simulink model "IEEE13_ltc"  (Simulink 8.5)
settings: Solver=ode5  SolverMode=SingleTasking  StartTime=0.0  StopTime=86400  FixedStep=Ts  RelTol=1e-3
PostLoadFcn:
  | Ts=3;
InitFcn:
  | Ts=3;
libraries: simulink x5, rtlab x1, rtlab_phasor x1
settings Model: Creator=GunaBharati  LastModifiedBy=Jaimie.Swartz
settings DataIOCC: SignalLoggingSaveFormat=Dataset  SaveOutput=off  SaveTime=off
settings OptimizationCC: BlockReduction=off  OptimizeBlockIOStorage=off  BufferReuse=off  GlobalBufferReuse=off  ExpressionFolding=off  ExpressionDepthLimit=128  LocalBlockOutputs=off
settings DebuggingCC: UnderspecifiedInitializationDetection=Simplified  MergeDetectMultiDrivingBlocksExec=error  FcnCallInpInsideContextMsg=EnableAllAsError  StateNameClashWarn=none
settings GRTTargetCC: CombineOutputUpdateFcns=on  GRTInterface=off
settings ConfigurationSet: Description=SimMechanics 2G

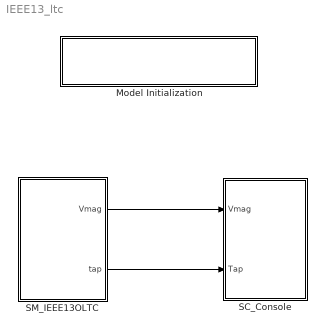
== system IEEE13_ltc ==
  Model Initialization : Subsystem  AncestorBlock=artemis/Tools /Misc/Model Initialization  mask(Model Functions){InitFcnX=Ts=3;, prel=off, posl=on, inif=on, strf=off}
      mask prompts: InitFcnX "Initialisation"; prel "Preload Function"; posl "PostLoad Function"; inif "InitFcn"; strf "StartFcn"
      mask init:
      | currentBlock = gcb;
      | root = bdroot(currentBlock);
      | 
      | if ~strcmp(get_param(root,'BlockDiagramType'),'library')
      |     if prel==1
      |         set_param(root, 'PreLoadFcn', InitFcnX);
      |     else
      |         set_param(root, 'PreLoadFcn', '');
      |     end
      |     if inif==1
      |         set_param(root, 'InitFcn', InitFcnX);
      |     else
      |         set_param(root, 'InitFcn', '');
      |     end
      |     if strf==1
      |         set_param(root, 'StartFcn', InitFcnX);
      |     else
      |         set_param(root, 'StartFcn', '');
      |     end
      |     if posl==1
      |         set_param(root, 'PostLoadFcn', InitFcnX);
      |     else
      |         set_param(root, 'PostLoadFcn', '');
      |     end
      | end
      | 
      | pos = get_param(currentBlock, 'Position');
      | width = pos(3) - pos(1); height = pos(4) - pos(2);
      | txt = [ upper(root) '\n' '- InitFcn. . . . . '  get_param(root, 'InitFcn') ];
      settings: CopyFcn=set_param(gcb,'LinkStatus','inactive')
      mask Display: text(5, height*0.5, txt, 'horizontalAlignment', 'left', 'verticalAlignment', 'middle') ;
  SC_Console : Subsystem
  SM_IEEE13OLTC : Subsystem
  wires:
  SM_IEEE13OLTC/1(Vmag) -> SC_Console/1(Vmag)
  SM_IEEE13OLTC/2(tap) -> SC_Console/2(Tap)

== system IEEE13_ltc/Model Initialization ==

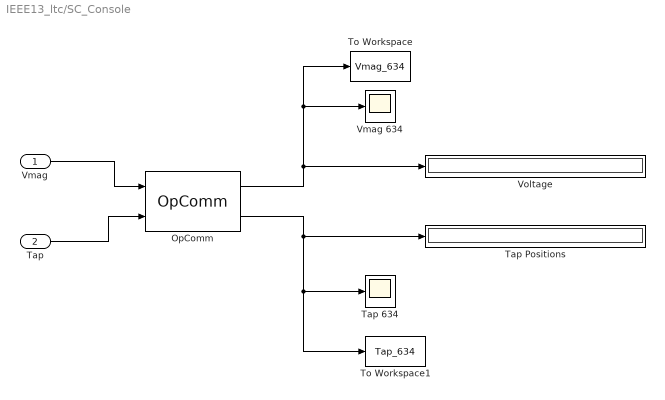
== system IEEE13_ltc/SC_Console ==
  Vmag : Inport
  Tap : Inport  Port=2
  OpComm : rtlab/OpComm  nbport=2  groupe_acq=1  subsys_rate=0  st=0  Synchronization=on  Interpolation=on  Threshold=1.0  Missed_Data=off  Sim_Time=off  Samples=off  dynSigOut=off  from_console=0  warning_done=off  writeOpCommFile=off  Offset=off
  Tap 634 : Scope
      settings: TimeRange=300  YMin=-1  YMax=1
  Tap Positions : Display
  To Workspace : ToWorkspace  VariableName=Vmag_634  SampleTime=-1
  To Workspace1 : ToWorkspace  VariableName=Tap_634  SampleTime=-1
  Vmag 634 : Scope
      settings: YMin=246.783  YMax=272.761
  Voltage : Display
  wires:
  Vmag/1 -> OpComm/1
  Tap/1 -> OpComm/2
  OpComm/1 -> Voltage/1, To Workspace/1, Vmag 634/1
  OpComm/2 -> Tap Positions/1, To Workspace1/1, Tap 634/1

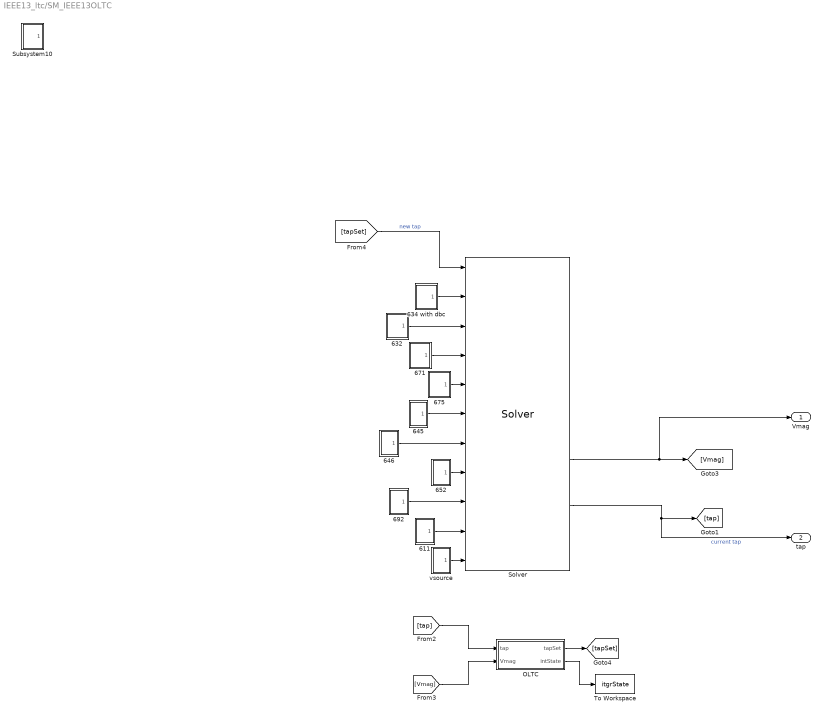
== system IEEE13_ltc/SM_IEEE13OLTC ==
  611 : Subsystem
  632 : Subsystem
  634 with dbc : Subsystem
  645 : Subsystem
  646 : Subsystem
  652 : Subsystem
  671 : Subsystem
  675 : Subsystem
  692 : Subsystem
  OLTC : Subsystem  mask{vRef=[260 260 260], intgConst=1200, deadBand=3.5/260, tapPos=[16 -16]}
      mask prompts: vRef "Reference Voltage: [a b c] voltage"; intgConst "Integrator Reset Value"; deadBand "Total Dead Band (pu)"; tapPos "[Max Min] Tap Positions"
      mask DialogControl DescTextVar Prompt: 3-Phase Voltage Regulator: Individual phase regulation enabled
  Solver : rtlab_phasor/Solver  epname=System  extension=Excel  xls='IEEE13_ltc_liz.xls'  raw='4992b.raw'  dyr='4992b.dyr'  cyme='typical.sxst'  powerfactory='network.dgs'  builtin=on  cyme_pf=''  cyme_unbalanced=on  lazy_netlist=off  capidir='CAPI'  fmudir=''  capiprefix=capicomp_  fmuprefix=fmucomp_  logging=off  sim_mode=Dynamic simulation only (without power-flow)  pf_max_it=100  pf_tol_v=0.00000001  pf_flat_start=off  pf_smart_start=off  pf_export=on  np=1  exporty=off  dt=Ts  optim_threads=on  perflog_on=off  script_activate_postinit=off  script_postinit_name=''
  Subsystem10 : Subsystem
  To Workspace : ToWorkspace  VariableName=itgrState  SampleTime=-1
  vsource : Subsystem
  Vmag : Outport
  tap : Outport  Port=2
  wires:
  Solver/5 -> Vmag/1, [Vmag]
  Solver/6 -> tap/1, [tap]  "current tap"
  OLTC/1(tapSet) -> [tapSet]
  [tapSet] -> Solver/1  "new tap"
  [Vmag] -> OLTC/2(Vmag)
  [tap] -> OLTC/1(tap)
  OLTC/2(intState) -> To Workspace/1
  632/1(Out1) -> Solver/3
  634 with dbc/1(Out1) -> Solver/2
  vsource/1(Out1) -> Solver/11
  611/1(Out1) -> Solver/10
  692/1(Out1) -> Solver/9
  652/1(Out1) -> Solver/8
  646/1(Out1) -> Solver/7
  645/1(Out1) -> Solver/6
  675/1(Out1) -> Solver/5
  671/1(Out1) -> Solver/4

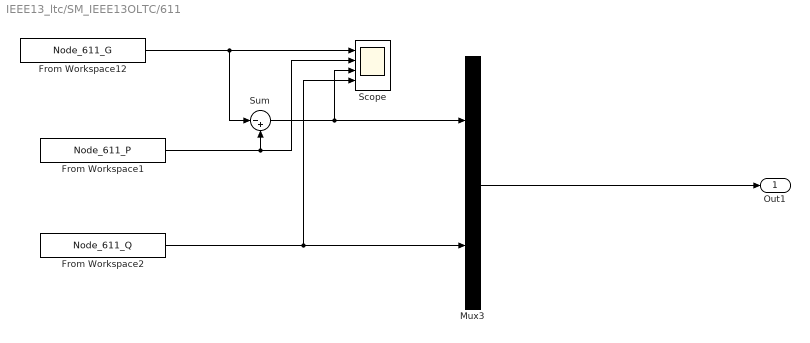
== system IEEE13_ltc/SM_IEEE13OLTC/611 ==
  From Workspace1 : FromWorkspace  VariableName=Node_611_P  SampleTime=Ts  OutputAfterFinalValue=Holding final value
  From Workspace12 : FromWorkspace  VariableName=Node_611_G  SampleTime=Ts  OutputAfterFinalValue=Holding final value
  From Workspace2 : FromWorkspace  VariableName=Node_611_Q  SampleTime=Ts  OutputAfterFinalValue=Holding final value
  Mux3 : Mux  Inputs=2
  Scope : Scope  NumInputPorts=4
      settings: YMin=229~-50~-5~-5  YMax=231~800~5~5  SampleInput=on  SampleTime=Ts
  Sum : Sum  Inputs=|-+
  Out1 : Outport
  wires:
  Mux3/1 -> Out1/1
  From Workspace2/1 -> Scope/4, Mux3/2
  From Workspace12/1 -> Sum/1, Scope/1
  Sum/1 -> Scope/3, Mux3/1
  From Workspace1/1 -> Sum/2, Scope/2

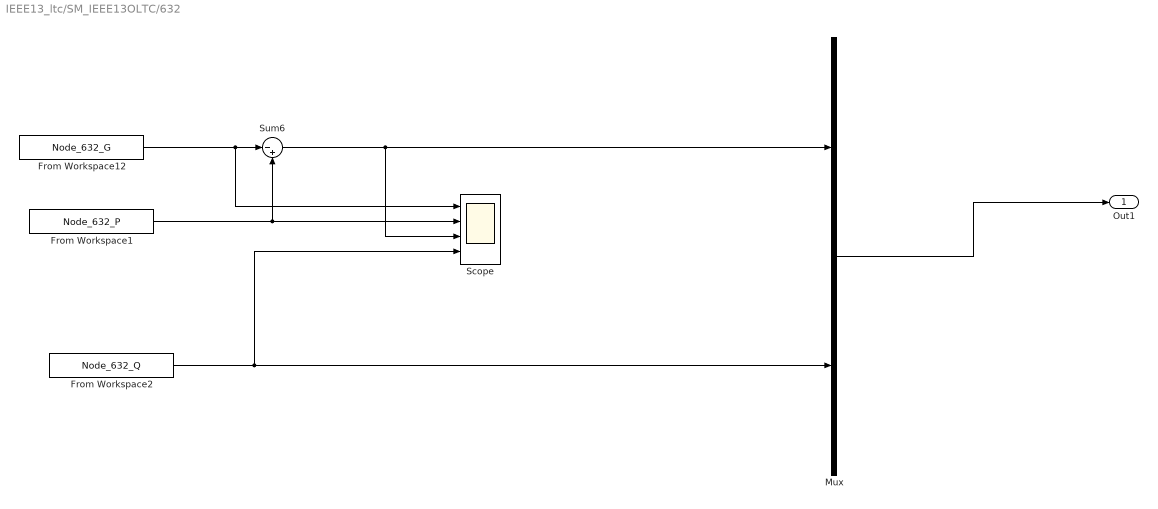
== system IEEE13_ltc/SM_IEEE13OLTC/632 ==
  From Workspace1 : FromWorkspace  VariableName=Node_632_P  SampleTime=Ts  OutputAfterFinalValue=Holding final value
  From Workspace12 : FromWorkspace  VariableName=Node_632_G  SampleTime=Ts  OutputAfterFinalValue=Holding final value
  From Workspace2 : FromWorkspace  VariableName=Node_632_Q  SampleTime=Ts  OutputAfterFinalValue=Holding final value
  Mux : Mux  Inputs=2
  Scope : Scope  NumInputPorts=4
      settings: YMin=229~-50~-5~-5  YMax=231~800~5~5  SaveName=ScopeData2  SampleInput=on  SampleTime=Ts
  Sum6 : Sum  Inputs=|-+
  Out1 : Outport
  wires:
  Mux/1 -> Out1/1
  From Workspace2/1 -> Mux/2, Scope/4
  From Workspace12/1 -> Scope/1, Sum6/1
  Sum6/1 -> Scope/3, Mux/1
  From Workspace1/1 -> Sum6/2, Scope/2

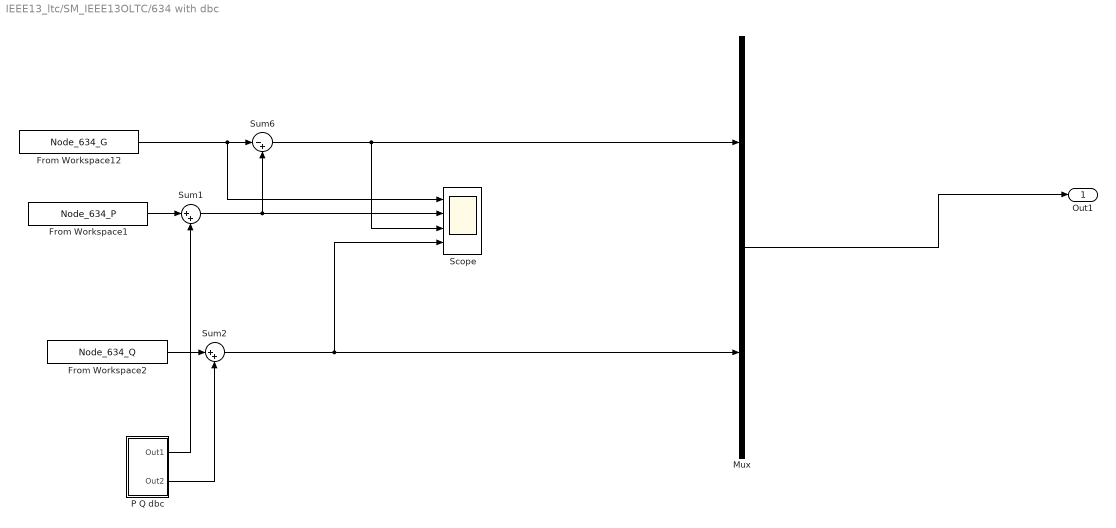
== system IEEE13_ltc/SM_IEEE13OLTC/634 with dbc ==
  From Workspace1 : FromWorkspace  VariableName=Node_634_P  SampleTime=Ts  OutputAfterFinalValue=Holding final value
  From Workspace12 : FromWorkspace  VariableName=Node_634_G  SampleTime=Ts  OutputAfterFinalValue=Holding final value
  From Workspace2 : FromWorkspace  VariableName=Node_634_Q  SampleTime=Ts  OutputAfterFinalValue=Holding final value
  Mux : Mux  Inputs=2
  P Q dbc : Subsystem
  Scope : Scope  NumInputPorts=4
      settings: YMin=229~-50~-5~-5  YMax=231~800~5~5  SaveName=ScopeData2  SampleInput=on  SampleTime=Ts
  Sum1 : Sum  Inputs=|++
  Sum2 : Sum  Inputs=|++
  Sum6 : Sum  Inputs=|-+
  Out1 : Outport
  wires:
  Mux/1 -> Out1/1
  From Workspace12/1 -> Scope/1, Sum6/1
  Sum6/1 -> Scope/3, Mux/1
  From Workspace1/1 -> Sum1/1
  Sum1/1 -> Sum6/2, Scope/2
  Sum2/1 -> Mux/2, Scope/4
  From Workspace2/1 -> Sum2/1
  P Q dbc/2(Out2) -> Sum2/2
  P Q dbc/1(Out1) -> Sum1/2

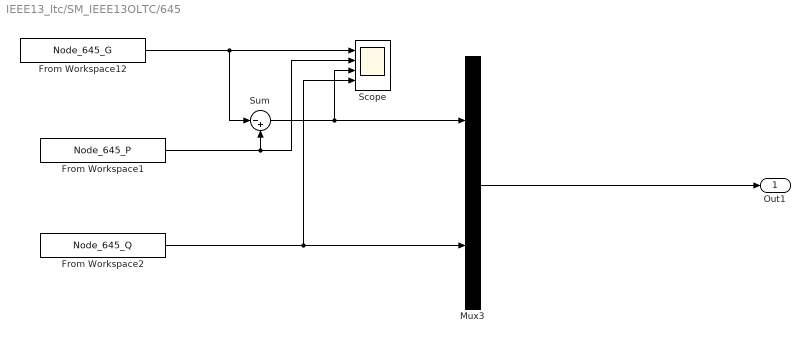
== system IEEE13_ltc/SM_IEEE13OLTC/645 ==
  From Workspace1 : FromWorkspace  VariableName=Node_645_P  SampleTime=Ts  OutputAfterFinalValue=Holding final value
  From Workspace12 : FromWorkspace  VariableName=Node_645_G  SampleTime=Ts  OutputAfterFinalValue=Holding final value
  From Workspace2 : FromWorkspace  VariableName=Node_645_Q  SampleTime=Ts  OutputAfterFinalValue=Holding final value
  Mux3 : Mux  Inputs=2
  Scope : Scope  NumInputPorts=4
      settings: YMin=229~-50~-5~-5  YMax=231~800~5~5  SampleInput=on  SampleTime=Ts
  Sum : Sum  Inputs=|-+
  Out1 : Outport
  wires:
  Mux3/1 -> Out1/1
  From Workspace2/1 -> Scope/4, Mux3/2
  From Workspace12/1 -> Sum/1, Scope/1
  Sum/1 -> Scope/3, Mux3/1
  From Workspace1/1 -> Sum/2, Scope/2

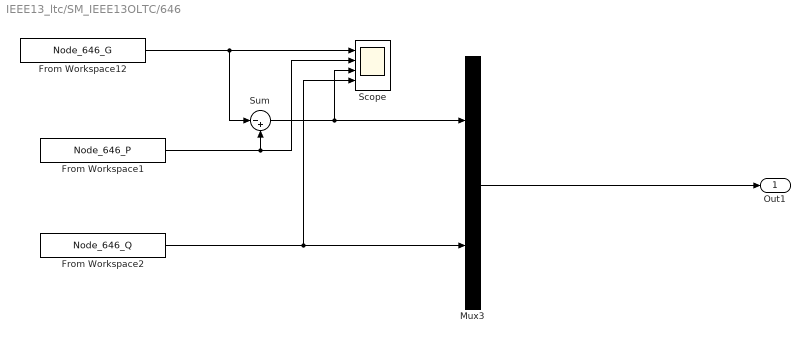
== system IEEE13_ltc/SM_IEEE13OLTC/646 ==
  From Workspace1 : FromWorkspace  VariableName=Node_646_P  SampleTime=Ts  OutputAfterFinalValue=Holding final value
  From Workspace12 : FromWorkspace  VariableName=Node_646_G  SampleTime=Ts  OutputAfterFinalValue=Holding final value
  From Workspace2 : FromWorkspace  VariableName=Node_646_Q  SampleTime=Ts  OutputAfterFinalValue=Holding final value
  Mux3 : Mux  Inputs=2
  Scope : Scope  NumInputPorts=4
      settings: YMin=229~-50~-5~-5  YMax=231~800~5~5  SampleInput=on  SampleTime=Ts
  Sum : Sum  Inputs=|-+
  Out1 : Outport
  wires:
  Mux3/1 -> Out1/1
  From Workspace2/1 -> Scope/4, Mux3/2
  From Workspace12/1 -> Sum/1, Scope/1
  Sum/1 -> Scope/3, Mux3/1
  From Workspace1/1 -> Sum/2, Scope/2

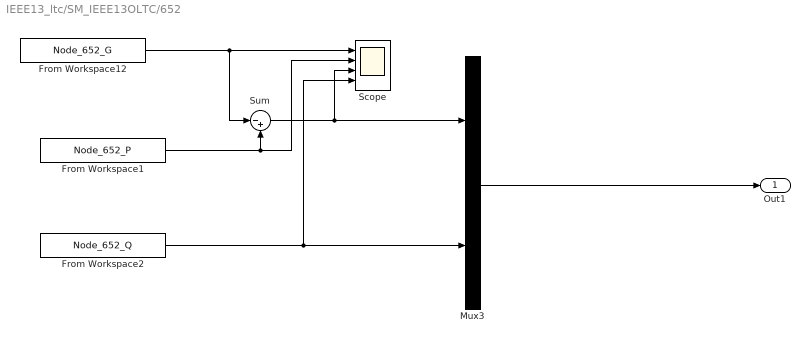
== system IEEE13_ltc/SM_IEEE13OLTC/652 ==
  From Workspace1 : FromWorkspace  VariableName=Node_652_P  SampleTime=Ts  OutputAfterFinalValue=Holding final value
  From Workspace12 : FromWorkspace  VariableName=Node_652_G  SampleTime=Ts  OutputAfterFinalValue=Holding final value
  From Workspace2 : FromWorkspace  VariableName=Node_652_Q  SampleTime=Ts  OutputAfterFinalValue=Holding final value
  Mux3 : Mux  Inputs=2
  Scope : Scope  NumInputPorts=4
      settings: YMin=229~-50~-5~-5  YMax=231~800~5~5  SampleInput=on  SampleTime=Ts
  Sum : Sum  Inputs=|-+
  Out1 : Outport
  wires:
  Mux3/1 -> Out1/1
  From Workspace2/1 -> Scope/4, Mux3/2
  From Workspace12/1 -> Sum/1, Scope/1
  Sum/1 -> Scope/3, Mux3/1
  From Workspace1/1 -> Sum/2, Scope/2

== system IEEE13_ltc/SM_IEEE13OLTC/671 ==
  From Workspace1 : FromWorkspace  VariableName=Node_671_P  SampleTime=Ts  OutputAfterFinalValue=Holding final value
  From Workspace12 : FromWorkspace  VariableName=Node_671_G  SampleTime=Ts  OutputAfterFinalValue=Holding final value
  From Workspace2 : FromWorkspace  VariableName=Node_671_Q  SampleTime=Ts  OutputAfterFinalValue=Holding final value
  Mux : Mux  Inputs=2
  Scope : Scope  NumInputPorts=4
      settings: YMin=229~-50~-5~-5  YMax=231~800~5~5  SaveName=ScopeData2  SampleInput=on  SampleTime=Ts
  Sum6 : Sum  Inputs=|-+
  Out1 : Outport
  wires:
  Mux/1 -> Out1/1
  From Workspace2/1 -> Mux/2, Scope/4
  From Workspace12/1 -> Scope/1, Sum6/1
  Sum6/1 -> Scope/3, Mux/1
  From Workspace1/1 -> Sum6/2, Scope/2

== system IEEE13_ltc/SM_IEEE13OLTC/675 ==
  From Workspace1 : FromWorkspace  VariableName=Node_675_P  SampleTime=Ts  OutputAfterFinalValue=Holding final value
  From Workspace12 : FromWorkspace  VariableName=Node_675_G  SampleTime=Ts  OutputAfterFinalValue=Holding final value
  From Workspace2 : FromWorkspace  VariableName=Node_675_Q  SampleTime=Ts  OutputAfterFinalValue=Holding final value
  Mux : Mux  Inputs=2
  Scope : Scope  NumInputPorts=4
      settings: YMin=229~-50~-5~-5  YMax=231~800~5~5  SaveName=ScopeData2  SampleInput=on  SampleTime=Ts
  Sum6 : Sum  Inputs=|-+
  Out1 : Outport
  wires:
  Mux/1 -> Out1/1
  From Workspace2/1 -> Mux/2, Scope/4
  From Workspace12/1 -> Scope/1, Sum6/1
  Sum6/1 -> Scope/3, Mux/1
  From Workspace1/1 -> Sum6/2, Scope/2

== system IEEE13_ltc/SM_IEEE13OLTC/692 ==
  From Workspace1 : FromWorkspace  VariableName=Node_692_P  SampleTime=Ts  OutputAfterFinalValue=Holding final value
  From Workspace12 : FromWorkspace  VariableName=Node_692_G  SampleTime=Ts  OutputAfterFinalValue=Holding final value
  From Workspace2 : FromWorkspace  VariableName=Node_692_Q  SampleTime=Ts  OutputAfterFinalValue=Holding final value
  Mux3 : Mux  Inputs=2
  Scope : Scope  NumInputPorts=4
      settings: YMin=229~-50~-5~-5  YMax=231~800~5~5  SampleInput=on  SampleTime=Ts
  Sum : Sum  Inputs=|-+
  Out1 : Outport
  wires:
  Mux3/1 -> Out1/1
  From Workspace2/1 -> Scope/4, Mux3/2
  From Workspace12/1 -> Sum/1, Scope/1
  Sum/1 -> Scope/3, Mux3/1
  From Workspace1/1 -> Sum/2, Scope/2

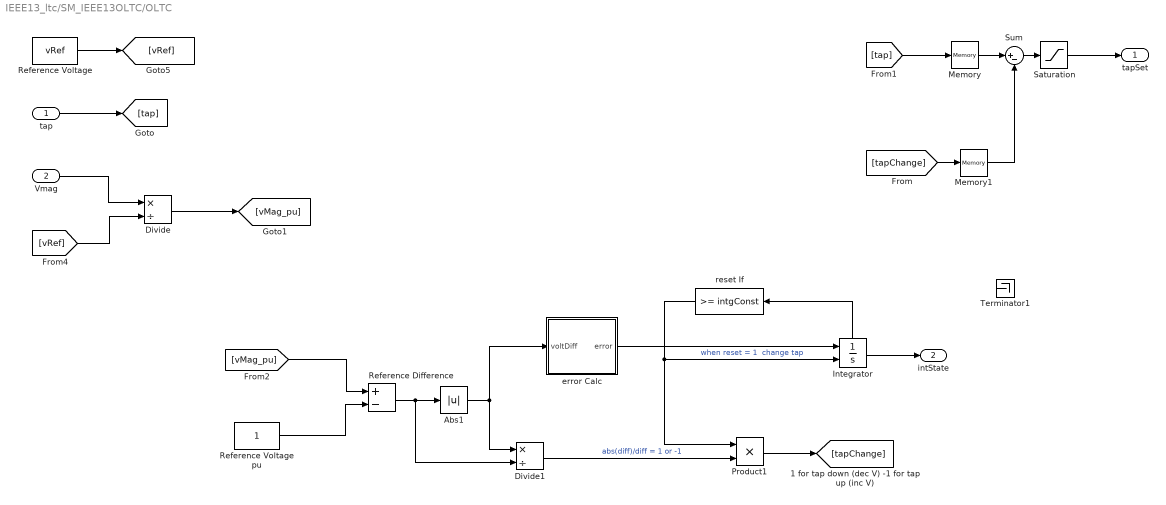
== system IEEE13_ltc/SM_IEEE13OLTC/OLTC ==
  tap : Inport
  Vmag : Inport  Port=2
  Abs1 : Abs
  Divide : Product  Inputs=*/
  Divide1 : Product  Inputs=*/
  Integrator : Integrator  ExternalReset=rising  ShowStatePort=on
  Memory : Memory
  Memory1 : Memory
  Product1 : Product
  Reference Difference : Sum  Inputs=+-
  Reference Voltage : Constant  Value=vRef
  Reference Voltage pu : Constant
  Saturation : Saturate  UpperLimit=tapPos(1)  LowerLimit=tapPos(2)
  Sum : Sum  Inputs=|+-
  Terminator1 : Terminator
  error Calc : Subsystem
  reset If : simulink/Logic and Bit Operations/Compare To Constant  relop=>=  const=intgConst  OutDataTypeStr=boolean
  tapSet : Outport
  intState : Outport  Port=2
  wires:
  Reference Voltage pu/1 -> Reference Difference/2
  Reference Difference/1 -> Divide1/2, Abs1/1
  Abs1/1 -> Divide1/1, error Calc/1(voltDiff)
  Divide1/1 -> Product1/2  "abs(diff)/diff = 1 or -1"
  Product1/1 -> [tapChange]
  Integrator/State -> reset If/1
  reset If/1 -> Product1/1, Integrator/2  "when reset = 1  change tap"
  [tap] -> Memory/1
  Sum/1 -> Saturation/1
  Memory/1 -> Sum/1
  [tapChange] -> Memory1/1
  Memory1/1 -> Sum/2
  tap/1 -> [tap]
  [vMag_pu] -> Reference Difference/1
  Saturation/1 -> tapSet/1
  Vmag/1 -> Divide/1
  Divide/1 -> [vMag_pu]
  [vRef] -> Divide/2
  Reference Voltage/1 -> [vRef]
  error Calc/1(error) -> Integrator/1
  Integrator/1 -> intState/1

== system IEEE13_ltc/SM_IEEE13OLTC/Subsystem10 ==
  From Workspace1 : FromWorkspace  VariableName=Node_634_P  SampleTime=Ts  OutputAfterFinalValue=Holding final value
  From Workspace12 : FromWorkspace  VariableName=Node_634_G  SampleTime=Ts  OutputAfterFinalValue=Holding final value
  From Workspace2 : FromWorkspace  VariableName=Node_634_Q  SampleTime=Ts  OutputAfterFinalValue=Holding final value
  Mux : Mux  Inputs=2
  Scope : Scope  NumInputPorts=4
      settings: YMin=229~-50~-5~-5  YMax=231~800~5~5  SaveName=ScopeData2  SampleInput=on  SampleTime=Ts
  Sum6 : Sum  Inputs=|-+
  Out1 : Outport
  wires:
  Mux/1 -> Out1/1
  From Workspace2/1 -> Mux/2, Scope/4
  From Workspace12/1 -> Scope/1, Sum6/1
  Sum6/1 -> Scope/3, Mux/1
  From Workspace1/1 -> Sum6/2, Scope/2

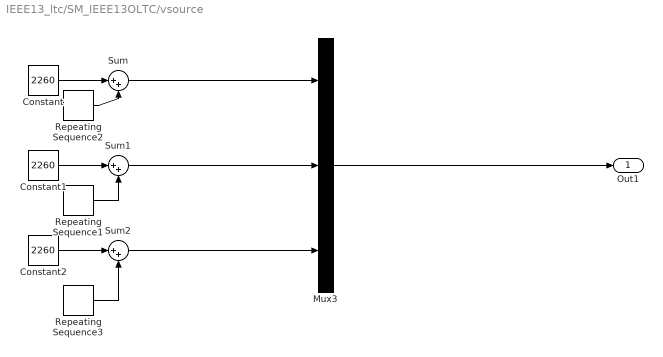
== system IEEE13_ltc/SM_IEEE13OLTC/vsource ==
  Constant : Constant  Value=2260
  Constant1 : Constant  Value=2260
  Constant2 : Constant  Value=2260
  Mux3 : Mux  Inputs=3
  Repeating Sequence1 : simulink/Sources/Repeating Sequence  rep_seq_t=[0 5000 10000 15000 20000 25000 30000 35000 40000 45000 50000 55000 60000 65000]  rep_seq_y="[0 10 20 30 40 50 60 50 40 30 20  15 10 5]"
  Repeating Sequence2 : simulink/Sources/Repeating Sequence  rep_seq_t=[0 5000 10000 15000 20000 25000 30000 35000 40000 45000 50000 55000 60000 65000]  rep_seq_y="[0 10 20 30 40 50 60 50 40 30 20  15 10 5]"
  Repeating Sequence3 : simulink/Sources/Repeating Sequence  rep_seq_t=[0 5000 10000 15000 20000 25000 30000 35000 40000 45000 50000 55000 60000 65000]  rep_seq_y="[0 10 20 30 40 50 60 50 40 30 20  15 10 5]"
  Sum : Sum  Inputs=|++
  Sum1 : Sum  Inputs=|++
  Sum2 : Sum  Inputs=|++
  Out1 : Outport
  wires:
  Mux3/1 -> Out1/1
  Constant/1 -> Sum/1
  Sum/1 -> Mux3/1
  Constant2/1 -> Sum2/1
  Constant1/1 -> Sum1/1
  Sum1/1 -> Mux3/2
  Sum2/1 -> Mux3/3
  Repeating Sequence3/1 -> Sum2/2
  Repeating Sequence1/1 -> Sum1/2
  Repeating Sequence2/1 -> Sum/2

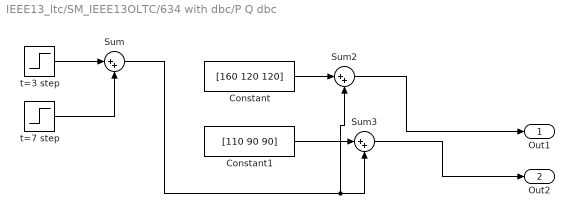
== system IEEE13_ltc/SM_IEEE13OLTC/634 with dbc/P Q dbc ==
  Constant : Constant  Value=[160 120 120]
  Constant1 : Constant  Value=[110 90 90]
  Sum : Sum  Inputs=|++
  Sum2 : Sum  Inputs=|++
  Sum3 : Sum  Inputs=|++
  t=3 step : Step  Time=3  After=100  SampleTime=0
  t=7 step : Step  Time=7  After=-200  SampleTime=0
  Out1 : Outport
  Out2 : Outport  Port=2
  wires:
  Constant/1 -> Sum2/1
  Sum/1 -> Sum3/2, Sum2/2
  Constant1/1 -> Sum3/1
  t=3 step/1 -> Sum/1
  Sum2/1 -> Out1/1
  t=7 step/1 -> Sum/2
  Sum3/1 -> Out2/1

== system IEEE13_ltc/SM_IEEE13OLTC/OLTC/error Calc ==
  note: if abs(voltage deviation from reference) is greater than 1/2 the deadband, error=1*dev
      | otherwise error=0*dev=0
  voltDiff : Inport
  Compare To Constant : simulink/Logic and Bit Operations/Compare To Constant  relop=>  const=0  OutDataTypeStr=boolean
  Gain : Gain  Gain=vRef
  Product : Product
  deadBand1 : Constant  Value=deadBand/2
  sub : Sum  Inputs=-+
  error : Outport
  wires:
  deadBand1/1 -> sub/1
  voltDiff/1 -> Product/2, sub/2
  sub/1 -> Compare To Constant/1
  Compare To Constant/1 -> Product/1
  Gain/1 -> error/1
  Product/1 -> Gain/1
